simulink model "exp4_1_step_response"  (R2024b)
settings: Solver=ode45  StartTime=0.0  StopTime=10  MaxStep=0.01  RelTol=1e-3
settings Model: Creator=1  LastModifiedBy=1

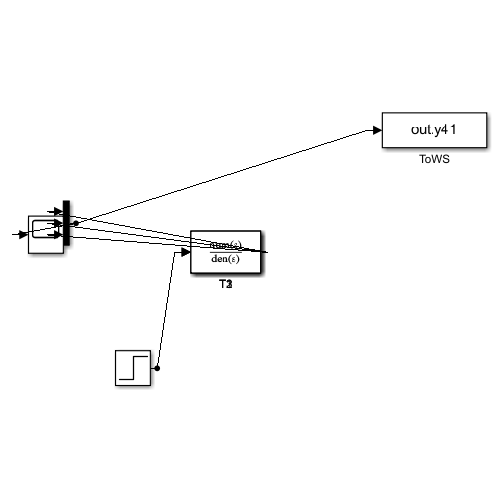
[thumbnail: Simulink's stored preview of the top-level diagram]
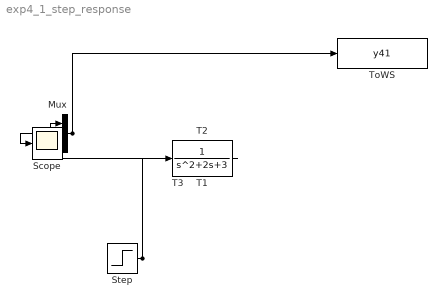
== system exp4_1_step_response ==
  Mux : Mux  Inputs=3
  Scope : Scope
  Step : Step  Time=0  SampleTime=0
  T1 : TransferFcn
  T2 : TransferFcn  Denominator=[1 2 2]
  T3 : TransferFcn  Denominator=[1 2 3]
  ToWS : ToWorkspace  VariableName=y41  SaveFormat=Timeseries  SampleTime=-1
  wires:
  Step/1 -> T1/1, T2/1, T3/1
  T1/1 -> Mux/1
  T2/1 -> Mux/2
  T3/1 -> Mux/3
  Mux/1 -> Scope/1, ToWS/1
